simulink model "case1"  (R2024b)
settings: Solver=FixedStepAuto  StartTime=0  StopTime=1  FixedStep=1e-7  RelTol=1e-3
values from neighbouring files (symbols this model uses):
  SG_D_1_D = 0.01056    [IEEE9_case_parameters.m]    (also in case1_parameters.m; case2_parameters.m; case3_parameters.m; case4_parameters.m)
  SG_D_1_EnableSaturation = 0    [IEEE9_case_parameters.m]    (also in case1_parameters.m; case2_parameters.m; case3_parameters.m; case4_parameters.m)
  SG_D_1_f0 = 60    [IEEE9_case_parameters.m]    (also in case1_parameters.m; case2_parameters.m; case3_parameters.m; case4_parameters.m)
  SG_D_1_H = 7.5    [IEEE9_case_parameters.m]    (also in case1_parameters.m; case2_parameters.m; case3_parameters.m; case4_parameters.m)
  SG_D_1_K_A = 20    [IEEE9_case_parameters.m]    (also in case1_parameters.m; case2_parameters.m; case3_parameters.m; case4_parameters.m)
  SG_D_1_K_E = 1.000000e+1    (= 10)    [IEEE9_case_parameters.m]    (also in case1_parameters.m; case2_parameters.m; case3_parameters.m; case4_parameters.m)
  SG_D_1_K_F = 2.363    [IEEE9_case_parameters.m]    (also in case1_parameters.m; case2_parameters.m; case3_parameters.m; case4_parameters.m)
  SG_D_1_K_s = 0.5    [IEEE9_case_parameters.m]    (also in case1_parameters.m = 5; case2_parameters.m = 5; case3_parameters.m = 5; case4_parameters.m = 5)
  SG_D_1_R_a = 0.001088    [IEEE9_case_parameters.m]    (also in case1_parameters.m; case2_parameters.m; case3_parameters.m; case4_parameters.m)
  SG_D_1_S_A = 1    [IEEE9_case_parameters.m]    (also in case1_parameters.m; case2_parameters.m; case3_parameters.m; case4_parameters.m)
  SG_D_1_S_B = 0.103    [IEEE9_case_parameters.m]    (also in case1_parameters.m; case2_parameters.m; case3_parameters.m; case4_parameters.m)
  SG_D_1_S_N = 10.659857    [IEEE9_case_parameters.m]    (also in case1_parameters.m; case2_parameters.m; case3_parameters.m; case4_parameters.m)
  SG_D_1_SpeedPara = 200    [IEEE9_case_parameters.m]    (also in case1_parameters.m; case2_parameters.m; case3_parameters.m; case4_parameters.m)
  SG_D_1_T_0 = 0.720173    [IEEE9_case_parameters.m]    (also in case1_parameters.m = 0.755522; case2_parameters.m = 0.808931; case3_parameters.m = 0.869402; case4_parameters.m = 0.729316)
  SG_D_1_T_1 = 0.3    [IEEE9_case_parameters.m]    (also in case1_parameters.m; case2_parameters.m; case3_parameters.m; case4_parameters.m)
  SG_D_1_T_2 = 0.05    [IEEE9_case_parameters.m]    (also in case1_parameters.m; case2_parameters.m; case3_parameters.m; case4_parameters.m)
  SG_D_1_T_3 = 0.02    [IEEE9_case_parameters.m]    (also in case1_parameters.m; case2_parameters.m; case3_parameters.m; case4_parameters.m)
  SG_D_1_T_4 = 0.005    [IEEE9_case_parameters.m]    (also in case1_parameters.m; case2_parameters.m; case3_parameters.m; case4_parameters.m)
  SG_D_1_T_A = 0.02    [IEEE9_case_parameters.m]    (also in case1_parameters.m; case2_parameters.m; case3_parameters.m; case4_parameters.m)
  SG_D_1_T_dd = 8.000000e+0    (= 8)    [IEEE9_case_parameters.m]    (also in case1_parameters.m; case2_parameters.m; case3_parameters.m; case4_parameters.m)
  SG_D_1_T_ddd = 0.04    [IEEE9_case_parameters.m]    (also in case1_parameters.m; case2_parameters.m; case3_parameters.m; case4_parameters.m)
  SG_D_1_T_E = 0.314    [IEEE9_case_parameters.m]    (also in case1_parameters.m; case2_parameters.m; case3_parameters.m; case4_parameters.m)
  SG_D_1_T_F = 0.35    [IEEE9_case_parameters.m]    (also in case1_parameters.m; case2_parameters.m; case3_parameters.m; case4_parameters.m)
  SG_D_1_T_qd = 0.8    [IEEE9_case_parameters.m]    (also in case1_parameters.m; case2_parameters.m; case3_parameters.m; case4_parameters.m)
  SG_D_1_T_qdd = 0.02    [IEEE9_case_parameters.m]    (also in case1_parameters.m; case2_parameters.m; case3_parameters.m; case4_parameters.m)
  SG_D_1_T_speed = 0.1    [IEEE9_case_parameters.m]    (also in case1_parameters.m = 200; case2_parameters.m = 200; case3_parameters.m = 200; case4_parameters.m = 200)
  SG_D_1_T_w = 0.5    [IEEE9_case_parameters.m]    (also in case1_parameters.m; case2_parameters.m; case3_parameters.m; case4_parameters.m)
  SG_D_1_V_ref = 1.990276    [IEEE9_case_parameters.m]    (also in case1_parameters.m = 2.042296; case2_parameters.m = 2.051388; case3_parameters.m = 2.089584; case4_parameters.m = 2.01845)
  SG_D_1_w_ref = 376.991118    [IEEE9_case_parameters.m]    (also in case1_parameters.m; case2_parameters.m; case3_parameters.m; case4_parameters.m)
  SG_D_1_wb = 6.000000e+1    (= 60)    [IEEE9_case_parameters.m]    (also in case1_parameters.m; case2_parameters.m; case3_parameters.m; case4_parameters.m)
  SG_D_1_x_d = 1.9    [IEEE9_case_parameters.m]    (also in case1_parameters.m; case2_parameters.m; case3_parameters.m; case4_parameters.m)
  SG_D_1_x_dd = 0.302    [IEEE9_case_parameters.m]    (also in case1_parameters.m; case2_parameters.m; case3_parameters.m; case4_parameters.m)
  SG_D_1_x_ddd = 0.204    [IEEE9_case_parameters.m]    (also in case1_parameters.m; case2_parameters.m; case3_parameters.m; case4_parameters.m)
  SG_D_1_x_l = 0.05    [IEEE9_case_parameters.m]    (also in case1_parameters.m; case2_parameters.m; case3_parameters.m; case4_parameters.m)
  SG_D_1_x_q = 1.3    [IEEE9_case_parameters.m]    (also in case1_parameters.m; case2_parameters.m; case3_parameters.m; case4_parameters.m)
  SG_D_1_x_qd = 0.5    [IEEE9_case_parameters.m]    (also in case1_parameters.m; case2_parameters.m; case3_parameters.m; case4_parameters.m)
  SG_D_1_x_qdd = 0.3    [IEEE9_case_parameters.m]    (also in case1_parameters.m; case2_parameters.m; case3_parameters.m; case4_parameters.m)
  SG_D_2_D = 0.02    [IEEE9_case_parameters.m]    (also in case1_parameters.m; case2_parameters.m; case3_parameters.m; case4_parameters.m)
  SG_D_2_EnableSaturation = 0    [IEEE9_case_parameters.m]    (also in case1_parameters.m; case2_parameters.m; case3_parameters.m; case4_parameters.m)
  SG_D_2_f0 = 60    [IEEE9_case_parameters.m]    (also in case1_parameters.m; case2_parameters.m; case3_parameters.m; case4_parameters.m)
  SG_D_2_H = 8.000000e+0    (= 8)    [IEEE9_case_parameters.m]    (also in case1_parameters.m; case2_parameters.m; case3_parameters.m; case4_parameters.m)
  SG_D_2_K_A = 20    [IEEE9_case_parameters.m]    (also in case1_parameters.m; case2_parameters.m; case3_parameters.m; case4_parameters.m)
  SG_D_2_K_E = 1.000000e+1    (= 10)    [IEEE9_case_parameters.m]    (also in case1_parameters.m; case2_parameters.m; case3_parameters.m; case4_parameters.m)
  SG_D_2_K_F = 2.363    [IEEE9_case_parameters.m]    (also in case1_parameters.m; case2_parameters.m; case3_parameters.m; case4_parameters.m)
  SG_D_2_K_s = 0.5    [IEEE9_case_parameters.m]    (also in case1_parameters.m = 4; case2_parameters.m = 4; case3_parameters.m = 4; case4_parameters.m = 4)
  SG_D_2_R_a = 0.001088    [IEEE9_case_parameters.m]    (also in case1_parameters.m; case2_parameters.m; case3_parameters.m; case4_parameters.m)
  SG_D_2_S_A = 1    [IEEE9_case_parameters.m]    (also in case1_parameters.m; case2_parameters.m; case3_parameters.m; case4_parameters.m)
  SG_D_2_S_B = 0.103    [IEEE9_case_parameters.m]    (also in case1_parameters.m; case2_parameters.m; case3_parameters.m; case4_parameters.m)
  SG_D_2_S_N = 10.659857    [IEEE9_case_parameters.m]    (also in case1_parameters.m; case2_parameters.m; case3_parameters.m; case4_parameters.m)
  SG_D_2_SpeedPara = 200    [IEEE9_case_parameters.m]    (also in case1_parameters.m; case2_parameters.m; case3_parameters.m; case4_parameters.m)
  SG_D_2_T_0 = 1.632913    [IEEE9_case_parameters.m]    (also in case1_parameters.m = 1.632925; case2_parameters.m = 1.632915; case3_parameters.m = 1.632914; case4_parameters.m = 1.632927)
  SG_D_2_T_1 = 0.2    [IEEE9_case_parameters.m]    (also in case1_parameters.m; case2_parameters.m; case3_parameters.m; case4_parameters.m)
  SG_D_2_T_2 = 0.05    [IEEE9_case_parameters.m]    (also in case1_parameters.m; case2_parameters.m; case3_parameters.m; case4_parameters.m)
  SG_D_2_T_3 = 0.02    [IEEE9_case_parameters.m]    (also in case1_parameters.m; case2_parameters.m; case3_parameters.m; case4_parameters.m)
  SG_D_2_T_4 = 0.005    [IEEE9_case_parameters.m]    (also in case1_parameters.m; case2_parameters.m; case3_parameters.m; case4_parameters.m)
  SG_D_2_T_A = 0.02    [IEEE9_case_parameters.m]    (also in case1_parameters.m; case2_parameters.m; case3_parameters.m; case4_parameters.m)
  SG_D_2_T_dd = 7.9    [IEEE9_case_parameters.m]    (also in case1_parameters.m; case2_parameters.m; case3_parameters.m; case4_parameters.m)
  SG_D_2_T_ddd = 0.04    [IEEE9_case_parameters.m]    (also in case1_parameters.m; case2_parameters.m; case3_parameters.m; case4_parameters.m)
  SG_D_2_T_E = 0.314    [IEEE9_case_parameters.m]    (also in case1_parameters.m; case2_parameters.m; case3_parameters.m; case4_parameters.m)
  SG_D_2_T_F = 0.35    [IEEE9_case_parameters.m]    (also in case1_parameters.m; case2_parameters.m; case3_parameters.m; case4_parameters.m)
  SG_D_2_T_qd = 0.8    [IEEE9_case_parameters.m]    (also in case1_parameters.m; case2_parameters.m; case3_parameters.m; case4_parameters.m)
  SG_D_2_T_qdd = 0.015    [IEEE9_case_parameters.m]    (also in case1_parameters.m; case2_parameters.m; case3_parameters.m; case4_parameters.m)
  SG_D_2_T_speed = 0.1    [IEEE9_case_parameters.m]    (also in case1_parameters.m = 150; case2_parameters.m = 150; case3_parameters.m = 150; case4_parameters.m = 150)
  SG_D_2_T_w = 0.35    [IEEE9_case_parameters.m]    (also in case1_parameters.m; case2_parameters.m; case3_parameters.m; case4_parameters.m)
  SG_D_2_V_ref = 2.58547    [IEEE9_case_parameters.m]    (also in case1_parameters.m = 2.597896; case2_parameters.m = 2.587136; case3_parameters.m = 2.586042; case4_parameters.m = 2.599679)
  SG_D_2_w_ref = 376.991118    [IEEE9_case_parameters.m]    (also in case1_parameters.m; case2_parameters.m; case3_parameters.m; case4_parameters.m)
  SG_D_2_wb = 6.000000e+1    (= 60)    [IEEE9_case_parameters.m]    (also in case1_parameters.m; case2_parameters.m; case3_parameters.m; case4_parameters.m)
  SG_D_2_x_d = 1.8    [IEEE9_case_parameters.m]    (also in case1_parameters.m; case2_parameters.m; case3_parameters.m; case4_parameters.m)
  SG_D_2_x_dd = 0.302    [IEEE9_case_parameters.m]    (also in case1_parameters.m; case2_parameters.m; case3_parameters.m; case4_parameters.m)
  SG_D_2_x_ddd = 0.204    [IEEE9_case_parameters.m]    (also in case1_parameters.m; case2_parameters.m; case3_parameters.m; case4_parameters.m)
  SG_D_2_x_l = 0.05    [IEEE9_case_parameters.m]    (also in case1_parameters.m; case2_parameters.m; case3_parameters.m; case4_parameters.m)
  SG_D_2_x_q = 1.25    [IEEE9_case_parameters.m]    (also in case1_parameters.m; case2_parameters.m; case3_parameters.m; case4_parameters.m)
  SG_D_2_x_qd = 0.5    [IEEE9_case_parameters.m]    (also in case1_parameters.m; case2_parameters.m; case3_parameters.m; case4_parameters.m)
  SG_D_2_x_qdd = 0.3    [IEEE9_case_parameters.m]    (also in case1_parameters.m; case2_parameters.m; case3_parameters.m; case4_parameters.m)
  SG_D_3_D = 0.02    [IEEE9_case_parameters.m]    (also in case1_parameters.m; case2_parameters.m; case3_parameters.m; case4_parameters.m)
  SG_D_3_EnableSaturation = 0    [IEEE9_case_parameters.m]    (also in case1_parameters.m; case2_parameters.m; case3_parameters.m; case4_parameters.m)
  SG_D_3_f0 = 60    [IEEE9_case_parameters.m]    (also in case1_parameters.m; case2_parameters.m; case3_parameters.m; case4_parameters.m)
  SG_D_3_H = 7.7    [IEEE9_case_parameters.m]    (also in case1_parameters.m; case2_parameters.m; case3_parameters.m; case4_parameters.m)
  SG_D_3_K_A = 20    [IEEE9_case_parameters.m]    (also in case1_parameters.m; case2_parameters.m; case3_parameters.m; case4_parameters.m)
  SG_D_3_K_E = 1.000000e+1    (= 10)    [IEEE9_case_parameters.m]    (also in case1_parameters.m; case2_parameters.m; case3_parameters.m; case4_parameters.m)
  SG_D_3_K_F = 2.363    [IEEE9_case_parameters.m]    (also in case1_parameters.m; case2_parameters.m; case3_parameters.m; case4_parameters.m)
  SG_D_3_K_s = 0.2    [IEEE9_case_parameters.m]    (also in case1_parameters.m = 2; case2_parameters.m = 2; case3_parameters.m = 2; case4_parameters.m = 2)
  SG_D_3_R_a = 0.001088    [IEEE9_case_parameters.m]    (also in case1_parameters.m; case2_parameters.m; case3_parameters.m; case4_parameters.m)
  SG_D_3_S_A = 1    [IEEE9_case_parameters.m]    (also in case1_parameters.m; case2_parameters.m; case3_parameters.m; case4_parameters.m)
  SG_D_3_S_B = 0.103    [IEEE9_case_parameters.m]    (also in case1_parameters.m; case2_parameters.m; case3_parameters.m; case4_parameters.m)
  SG_D_3_S_N = 10.659857    [IEEE9_case_parameters.m]    (also in case1_parameters.m; case2_parameters.m; case3_parameters.m; case4_parameters.m)
  SG_D_3_SpeedPara = 200    [IEEE9_case_parameters.m]    (also in case1_parameters.m; case2_parameters.m; case3_parameters.m; case4_parameters.m)
  SG_D_3_T_0 = 0.850788    [IEEE9_case_parameters.m]    (also in case1_parameters.m = 0.850786; case2_parameters.m = 0.850787; case3_parameters.m; case4_parameters.m = 0.850786)
  SG_D_3_T_1 = 0.2    [IEEE9_case_parameters.m]    (also in case1_parameters.m; case2_parameters.m; case3_parameters.m; case4_parameters.m)
  SG_D_3_T_2 = 0.05    [IEEE9_case_parameters.m]    (also in case1_parameters.m; case2_parameters.m; case3_parameters.m; case4_parameters.m)
  SG_D_3_T_3 = 0.02    [IEEE9_case_parameters.m]    (also in case1_parameters.m; case2_parameters.m; case3_parameters.m; case4_parameters.m)
  SG_D_3_T_4 = 0.005    [IEEE9_case_parameters.m]    (also in case1_parameters.m; case2_parameters.m; case3_parameters.m; case4_parameters.m)
  SG_D_3_T_A = 0.02    [IEEE9_case_parameters.m]    (also in case1_parameters.m; case2_parameters.m; case3_parameters.m; case4_parameters.m)
  SG_D_3_T_dd = 8.1    [IEEE9_case_parameters.m]    (also in case1_parameters.m; case2_parameters.m; case3_parameters.m; case4_parameters.m)
  SG_D_3_T_ddd = 0.04    [IEEE9_case_parameters.m]    (also in case1_parameters.m; case2_parameters.m; case3_parameters.m; case4_parameters.m)
  SG_D_3_T_E = 0.314    [IEEE9_case_parameters.m]    (also in case1_parameters.m; case2_parameters.m; case3_parameters.m; case4_parameters.m)
  SG_D_3_T_F = 0.35    [IEEE9_case_parameters.m]    (also in case1_parameters.m; case2_parameters.m; case3_parameters.m; case4_parameters.m)
  SG_D_3_T_qd = 0.8    [IEEE9_case_parameters.m]    (also in case1_parameters.m; case2_parameters.m; case3_parameters.m; case4_parameters.m)
  SG_D_3_T_qdd = 0.015    [IEEE9_case_parameters.m]    (also in case1_parameters.m; case2_parameters.m; case3_parameters.m; case4_parameters.m)
  SG_D_3_T_speed = 0.1    [IEEE9_case_parameters.m]    (also in case1_parameters.m = 180; case2_parameters.m = 180; case3_parameters.m = 180; case4_parameters.m = 180)
  SG_D_3_T_w = 0.4    [IEEE9_case_parameters.m]    (also in case1_parameters.m; case2_parameters.m; case3_parameters.m; case4_parameters.m)
  SG_D_3_V_ref = 1.892727    [IEEE9_case_parameters.m]    (also in case1_parameters.m = 1.906439; case2_parameters.m = 1.895535; case3_parameters.m = 1.892105; case4_parameters.m = 1.906598)
  SG_D_3_w_ref = 376.991118    [IEEE9_case_parameters.m]    (also in case1_parameters.m; case2_parameters.m; case3_parameters.m; case4_parameters.m)
  SG_D_3_wb = 6.000000e+1    (= 60)    [IEEE9_case_parameters.m]    (also in case1_parameters.m; case2_parameters.m; case3_parameters.m; case4_parameters.m)
  SG_D_3_x_d = 1.85    [IEEE9_case_parameters.m]    (also in case1_parameters.m; case2_parameters.m; case3_parameters.m; case4_parameters.m)
  SG_D_3_x_dd = 0.302    [IEEE9_case_parameters.m]    (also in case1_parameters.m; case2_parameters.m; case3_parameters.m; case4_parameters.m)
  SG_D_3_x_ddd = 0.204    [IEEE9_case_parameters.m]    (also in case1_parameters.m; case2_parameters.m; case3_parameters.m; case4_parameters.m)
  SG_D_3_x_l = 0.05    [IEEE9_case_parameters.m]    (also in case1_parameters.m; case2_parameters.m; case3_parameters.m; case4_parameters.m)
  SG_D_3_x_q = 1.2    [IEEE9_case_parameters.m]    (also in case1_parameters.m; case2_parameters.m; case3_parameters.m; case4_parameters.m)
  SG_D_3_x_qd = 0.5    [IEEE9_case_parameters.m]    (also in case1_parameters.m; case2_parameters.m; case3_parameters.m; case4_parameters.m)
  SG_D_3_x_qdd = 0.3    [IEEE9_case_parameters.m]    (also in case1_parameters.m; case2_parameters.m; case3_parameters.m; case4_parameters.m)
(part 10 of 12)

== system case1/SG_D_3/d_R_f_SG_D_3_block ==
  note: d_R_f_SG_D_3 in case1
      | $-\frac{R_{f,\mathrm{SG},D,3}-\frac{E_{\mathrm{fd},\mathrm{SG},D,3}\,K_{F}}{T_{F}}}{T_{F}}$
      | Automatically generated on 2025-10-31 18:49:57 .
  State_E_fd_SG_D_3_666b5 : Inport
  State_R_f_SG_D_3_7f0e0 : Inport  Port=2
  Constant_K_F_3ac82 : Constant  Value=K_F
  Constant_T_F_aca80 : Constant  Value=T_F
  Constant_T_F_d3988 : Constant  Value=T_F
  Divide_c9ce7 : Product  Inputs=*/
  Divide_de91c : Product  Inputs=*/
  Product_63f86 : Product
  Subtract_163d8 : Sum  Inputs=+-
  Blockout_d_R_f_SG_D_3_113ff : Outport
  wires:
  State_E_fd_SG_D_3_666b5/1 -> Product_63f86/1
  Constant_T_F_d3988/1 -> Divide_c9ce7/2
  Constant_K_F_3ac82/1 -> Product_63f86/2
  Product_63f86/1 -> Divide_c9ce7/1
  Divide_c9ce7/1 -> Subtract_163d8/1
  State_R_f_SG_D_3_7f0e0/1 -> Subtract_163d8/2
  Subtract_163d8/1 -> Divide_de91c/1
  Constant_T_F_aca80/1 -> Divide_de91c/2
  Divide_de91c/1 -> Blockout_d_R_f_SG_D_3_113ff/1

== system case1/SG_D_3/d_T_m_SG_D_3_block ==
  note: d_T_m_SG_D_3 in case1
      | $-\frac{T_{m,\mathrm{SG},D,3}-T_{0}+\frac{\mathrm{SpeedPara}\,\left(w_{\mathrm{SG},D,3}-w_{\mathrm{ref}}\right)}{2\,f_{0}\,\pi }}{T_{\mathrm{speed}}}$
      | Automatically generated on 2025-10-31 18:49:52 .
  State_w_SG_D_3_66142 : Inport
  State_T_m_SG_D_3_24b45 : Inport  Port=2
  Add_9f440 : Sum
  Add_ee289 : Sum
  Constant_-1_aa800 : Constant  Value=-1
  Constant_2.0_3da56 : Constant  Value=2.0
  Constant_SpeedPara_331ce : Constant  Value=SpeedPara
  Constant_T_0_ffd13 : Constant  Value=T_0
  Constant_T_speed_afd64 : Constant  Value=T_speed
  Constant_f0_5ced1 : Constant  Value=f0
  Constant_pi_16505 : Constant  Value=pi
  Constant_w_ref_a248d : Constant  Value=w_ref
  Divide_01cbf : Product  Inputs=*/
  Divide_61cdb : Product  Inputs=*/
  Product_7fe71 : Product
  Product_98dfd : Product
  Product_bc562 : Product
  Product_c22a6 : Product
  Subtract_d9e42 : Sum  Inputs=+-
  Blockout_d_T_m_SG_D_3_67a05 : Outport
  wires:
  Constant_SpeedPara_331ce/1 -> Product_7fe71/1
  Constant_-1_aa800/1 -> Product_98dfd/1
  Constant_w_ref_a248d/1 -> Add_9f440/2
  State_w_SG_D_3_66142/1 -> Product_98dfd/2
  Constant_2.0_3da56/1 -> Product_c22a6/1
  Product_98dfd/1 -> Add_9f440/1
  Constant_pi_16505/1 -> Product_c22a6/2
  Add_9f440/1 -> Product_7fe71/2
  Product_c22a6/1 -> Product_bc562/1
  Constant_f0_5ced1/1 -> Product_bc562/2
  Product_7fe71/1 -> Divide_01cbf/1
  Product_bc562/1 -> Divide_01cbf/2
  Divide_01cbf/1 -> Add_ee289/1
  Constant_T_0_ffd13/1 -> Add_ee289/2
  Add_ee289/1 -> Subtract_d9e42/1
  State_T_m_SG_D_3_24b45/1 -> Subtract_d9e42/2
  Subtract_d9e42/1 -> Divide_61cdb/1
  Constant_T_speed_afd64/1 -> Divide_61cdb/2
  Divide_61cdb/1 -> Blockout_d_T_m_SG_D_3_67a05/1

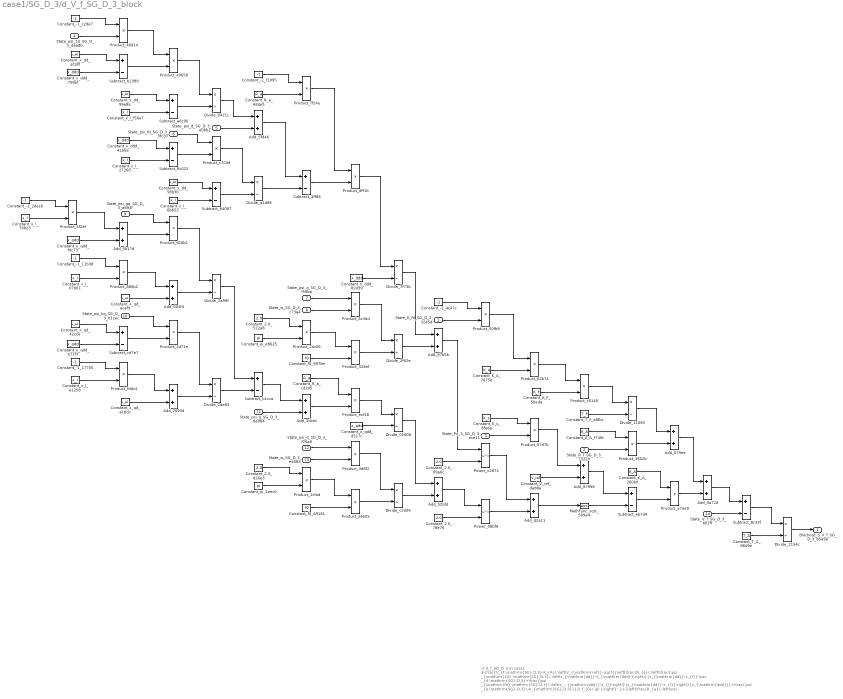
== system case1/SG_D_3/d_V_f_SG_D_3_block ==
  note: d_V_f_SG_D_3 in case1
      | $-\frac{V_{f,\mathrm{SG},D,3}-K_{A}\,\left(V_{\mathrm{ref}}-\sqrt{{\left(\frac{R_{a}\,\left(\frac{\psi _{\mathrm{1d},\mathrm{SG},D,3}\,\left(x_{\mathrm{dd}}-x_{\mathrm{ddd}}\right)}{x_{\mathrm{dd}}-x_{l}}-\psi _{d,\mathrm{SG},D,3}+\frac{\psi _{\mathrm{fd},\mathrm{SG},D,3}\,\left(x_{\mathrm{ddd}}-x_{l}\right)}{x_{\mathrm{dd}}-x_{l}}\right)}{x_{\mathrm{ddd}}}+\frac{\psi _{q,\mathrm{SG},D,3}\,w_{\mathrm{SG},D,3}}{2\,f_{0}\,\pi }\right)}^2+{\left(\frac{R_{a}\,\left(\psi _{q,\mathrm{SG},D,3}+\frac{\psi _{\mathrm{gq},\mathrm{SG},D,3}\,\left(x_{l}-x_{\mathrm{qdd}}\right)}{x_{l}-x_{\mathrm{qd}}}+\frac{\psi _{\mathrm{kq},\mathrm{SG},D,3}\,\left(x_{\mathrm{qd}}-x_{\mathrm{qdd}}\right)}{x_{l}-x_{\mathrm{qd}}}\right)}{x_{\mathrm{qdd}}}+\frac{\psi _{d,\mathrm{SG},D,3}\,w_{\mathrm{SG},D,3}}{2\,f_{0}\,\pi }\right)}^2}+K_{s}\,\mathrm{Px}_{3,\mathrm{SG},D,3}\right)-K_{A}\,R_{f,\mathrm{SG},D,3}+\frac{E_{\mathrm{fd},\mathrm{SG},D,3}\,K_{A}\,K_{F}}{T_{F}}}{T_{A}}$
      | Automatically generated on 2025-10-31 18:49:56 .
  State_E_fd_SG_D_3_3245d : Inport
  State_R_f_SG_D_3_73220 : Inport  Port=2
  State_Px_3_SG_D_3_ece11 : Inport  Port=3
  State_psi_1d_SG_D_3_daa8b : Inport  Port=4
  State_psi_d_SG_D_3_e0bb1 : Inport  Port=5
  State_psi_fd_SG_D_3_3fc20 : Inport  Port=6
  State_psi_q_SG_D_3_f59ba : Inport  Port=7
  State_w_SG_D_3_c73a4 : Inport  Port=8
  State_psi_gq_SG_D_3_a694f : Inport  Port=9
  State_psi_kq_SG_D_3_b1cec : Inport  Port=10
  State_psi_q_SG_D_3_dedb4 : Inport  Port=11
  State_psi_d_SG_D_3_f76a9 : Inport  Port=12
  State_w_SG_D_3_e4083 : Inport  Port=13
  State_V_f_SG_D_3_b01ff : Inport  Port=14
  Add_079ee : Sum
  Add_0a72d : Sum
  Add_2093d : Sum
  Add_3dcec : Sum
  Add_52bfd : Sum
  Add_5b17d : Sum
  Add_5fd46 : Sum
  Add_604f4 : Sum
  Add_87996 : Sum
  Add_97b5b : Sum
  Add_d2a11 : Sum
  Constant_-1_11b38 : Constant  Value=-1
  Constant_-1_17705 : Constant  Value=-1
  Constant_-1_2decb : Constant  Value=-1
  Constant_-1_4c47c : Constant  Value=-1
  Constant_-1_c29e7 : Constant  Value=-1
  Constant_-1_f1995 : Constant  Value=-1
  Constant_2.0_09a6c : Constant  Value=2.0
  Constant_2.0_522a8 : Constant  Value=2.0
  Constant_2.0_78e76 : Constant  Value=2.0
  Constant_2.0_d26e3 : Constant  Value=2.0
  Constant_K_A_260b0 : Constant  Value=K_A
  Constant_K_A_7675b : Constant  Value=K_A
  Constant_K_A_f74fe : Constant  Value=K_A
  Constant_K_F_50eda : Constant  Value=K_F
  Constant_K_s_8fe6a : Constant  Value=K_s
  Constant_R_a_68de5 : Constant  Value=R_a
  Constant_R_a_cd2d5 : Constant  Value=R_a
  Constant_T_A_8849e : Constant  Value=T_A
  Constant_T_F_af8bc : Constant  Value=T_F
  Constant_V_ref_da88a : Constant  Value=V_ref
  Constant_f0_69181 : Constant  Value=f0
  Constant_f0_9978e : Constant  Value=f0
  Constant_pi_1eec0 : Constant  Value=pi
  Constant_pi_e8625 : Constant  Value=pi
  Constant_x_dd_58b30 : Constant  Value=x_dd
  Constant_x_dd_99e8a : Constant  Value=x_dd
  Constant_x_dd_af18f : Constant  Value=x_dd
  Constant_x_ddd_41b5a : Constant  Value=x_ddd
  Constant_x_ddd_758ef : Constant  Value=x_ddd
  Constant_x_ddd_82d39 : Constant  Value=x_ddd
  Constant_x_l_07001 : Constant  Value=x_l
  Constant_x_l_27260 : Constant  Value=x_l
  Constant_x_l_6b652 : Constant  Value=x_l
  Constant_x_l_79823 : Constant  Value=x_l
  Constant_x_l_e1258 : Constant  Value=x_l
  Constant_x_l_f56a7 : Constant  Value=x_l
  Constant_x_qd_42cce : Constant  Value=x_qd
  Constant_x_qd_a18cb : Constant  Value=x_qd
  Constant_x_qd_acaf9 : Constant  Value=x_qd
  Constant_x_qdd_d517c : Constant  Value=x_qdd
  Constant_x_qdd_e71f3 : Constant  Value=x_qdd
  Constant_x_qdd_fdc73 : Constant  Value=x_qdd
  Divide_01608 : Product  Inputs=*/
  Divide_11083 : Product  Inputs=*/
  Divide_2154c : Product  Inputs=*/
  Divide_2a99f : Product  Inputs=*/
  Divide_2de83 : Product  Inputs=*/
  Divide_2f62e : Product  Inputs=*/
  Divide_7f73b : Product  Inputs=*/
  Divide_9421c : Product  Inputs=*/
  Divide_a1d88 : Product  Inputs=*/
  Divide_c2d09 : Product  Inputs=*/
  MathFunc_sqrt_599a4 : Sqrt
  Power_08bf6 : Math  Operator=pow
  Power_c2873 : Math  Operator=pow
  Product_1cfad : Product
  Product_26a05 : Product
  Product_2d71e : Product
  Product_2dc06 : Product
  Product_328ef : Product
  Product_3802b : Product
  Product_3d8f2 : Product
  Product_46914 : Product
  Product_4f2af : Product
  Product_50fb9 : Product
  Product_62b74 : Product
  Product_67d7b : Product
  Product_6c3dd : Product
  Product_880b2 : Product
  Product_a0658 : Product
  Product_a7ae9 : Product
  Product_c0148 : Product
  Product_c703d : Product
  Product_d16b1 : Product
  Product_dff1b : Product
  Product_ecf18 : Product
  Product_fddc4 : Product
  Product_ff24e : Product
  Subtract_4ff88 : Sum  Inputs=+-
  Subtract_64097 : Sum  Inputs=+-
  Subtract_8c022 : Sum  Inputs=+-
  Subtract_8c33f : Sum  Inputs=+-
  Subtract_a6c00 : Sum  Inputs=+-
  Subtract_b1cca : Sum  Inputs=+-
  Subtract_b2389 : Sum  Inputs=+-
  Subtract_cd7e7 : Sum  Inputs=+-
  Subtract_eb7d4 : Sum  Inputs=+-
  Blockout_d_V_f_SG_D_3_85a9a : Outport
  wires:
  Constant_K_A_f74fe/1 -> Product_3802b/1
  Constant_-1_2decb/1 -> Product_4f2af/1
  Subtract_8c022/1 -> Product_c703d/2
  Constant_x_l_79823/1 -> Product_4f2af/2
  Divide_c2d09/1 -> Add_52bfd/2
  Constant_-1_c29e7/1 -> Product_46914/1
  State_psi_1d_SG_D_3_daa8b/1 -> Product_46914/2
  Constant_x_dd_af18f/1 -> Subtract_b2389/1
  Divide_a1d88/1 -> Subtract_4ff88/2
  Product_4f2af/1 -> Add_5b17d/1
  Constant_x_qdd_fdc73/1 -> Add_5b17d/2
  Constant_x_ddd_758ef/1 -> Subtract_b2389/2
  Constant_2.0_78e76/1 -> Power_08bf6/2
  Constant_-1_11b38/1 -> Product_880b2/1
  Divide_2a99f/1 -> Subtract_b1cca/1
  Subtract_a6c00/1 -> Divide_9421c/2
  Constant_x_l_07001/1 -> Product_880b2/2
  Constant_x_qd_42cce/1 -> Subtract_cd7e7/1
  State_w_SG_D_3_c73a4/1 -> Product_6c3dd/2
  Constant_x_qdd_e71f3/1 -> Subtract_cd7e7/2
  Constant_2.0_522a8/1 -> Product_2dc06/1
  Constant_-1_17705/1 -> Product_fddc4/1
  Constant_pi_e8625/1 -> Product_2dc06/2
  Add_5fd46/1 -> Subtract_4ff88/1
  Constant_x_l_e1258/1 -> Product_fddc4/2
  Product_46914/1 -> Product_a0658/1
  Subtract_b2389/1 -> Product_a0658/2
  Constant_2.0_d26e3/1 -> Product_1cfad/1
  Constant_x_dd_99e8a/1 -> Subtract_a6c00/1
  Constant_pi_1eec0/1 -> Product_1cfad/2
  Constant_x_l_f56a7/1 -> Subtract_a6c00/2
  Constant_x_ddd_41b5a/1 -> Subtract_8c022/1
  Constant_x_l_27260/1 -> Subtract_8c022/2
  State_psi_gq_SG_D_3_a694f/1 -> Product_d16b1/1
  Constant_x_l_6b652/1 -> Subtract_64097/2
  Add_5b17d/1 -> Product_d16b1/2
  Product_880b2/1 -> Add_604f4/1
  Product_d16b1/1 -> Divide_2a99f/1
  Constant_x_qd_acaf9/1 -> Add_604f4/2
  State_psi_kq_SG_D_3_b1cec/1 -> Product_2d71e/1
  State_psi_q_SG_D_3_f59ba/1 -> Product_6c3dd/1
  Add_97b5b/1 -> Power_c2873/1
  Subtract_cd7e7/1 -> Product_2d71e/2
  Constant_f0_9978e/1 -> Product_328ef/2
  Product_2dc06/1 -> Product_328ef/1
  Constant_x_qd_a18cb/1 -> Add_2093d/2
  Product_fddc4/1 -> Add_2093d/1
  Product_a0658/1 -> Divide_9421c/1
  State_psi_fd_SG_D_3_3fc20/1 -> Product_c703d/1
  Constant_x_dd_58b30/1 -> Subtract_64097/1
  Add_604f4/1 -> Divide_2a99f/2
  Add_d2a11/1 -> MathFunc_sqrt_599a4/1
  Product_2d71e/1 -> Divide_2de83/1
  Add_2093d/1 -> Divide_2de83/2
  Product_ff24e/1 -> Product_dff1b/1
  Divide_9421c/1 -> Add_5fd46/1
  Add_87996/1 -> Subtract_eb7d4/1
  State_psi_d_SG_D_3_e0bb1/1 -> Add_5fd46/2
  Product_c703d/1 -> Divide_a1d88/1
  Subtract_64097/1 -> Divide_a1d88/2
  MathFunc_sqrt_599a4/1 -> Subtract_eb7d4/2
  Divide_2de83/1 -> Subtract_b1cca/2
  Constant_-1_f1995/1 -> Product_ff24e/1
  Constant_R_a_68de5/1 -> Product_ff24e/2
  Subtract_b1cca/1 -> Add_3dcec/1
  State_psi_q_SG_D_3_dedb4/1 -> Add_3dcec/2
  Subtract_4ff88/1 -> Product_dff1b/2
  Constant_R_a_cd2d5/1 -> Product_ecf18/1
  Add_3dcec/1 -> Product_ecf18/2
  State_psi_d_SG_D_3_f76a9/1 -> Product_3d8f2/1
  State_w_SG_D_3_e4083/1 -> Product_3d8f2/2
  Product_1cfad/1 -> Product_26a05/1
  Constant_f0_69181/1 -> Product_26a05/2
  Product_dff1b/1 -> Divide_7f73b/1
  Constant_x_ddd_82d39/1 -> Divide_7f73b/2
  Product_6c3dd/1 -> Divide_2f62e/1
  Product_328ef/1 -> Divide_2f62e/2
  Product_ecf18/1 -> Divide_01608/1
  Constant_x_qdd_d517c/1 -> Divide_01608/2
  Product_3d8f2/1 -> Divide_c2d09/1
  Product_26a05/1 -> Divide_c2d09/2
  Divide_7f73b/1 -> Add_97b5b/1
  Divide_2f62e/1 -> Add_97b5b/2
  Divide_01608/1 -> Add_52bfd/1
  Constant_-1_4c47c/1 -> Product_50fb9/1
  State_E_fd_SG_D_3_3245d/1 -> Product_50fb9/2
  Constant_2.0_09a6c/1 -> Power_c2873/2
  Add_52bfd/1 -> Power_08bf6/1
  Product_50fb9/1 -> Product_62b74/1
  Constant_K_A_7675b/1 -> Product_62b74/2
  Constant_K_s_8fe6a/1 -> Product_67d7b/1
  State_Px_3_SG_D_3_ece11/1 -> Product_67d7b/2
  Power_c2873/1 -> Add_d2a11/1
  Power_08bf6/1 -> Add_d2a11/2
  Product_62b74/1 -> Product_c0148/1
  Constant_K_F_50eda/1 -> Product_c0148/2
  Product_67d7b/1 -> Add_87996/1
  Constant_V_ref_da88a/1 -> Add_87996/2
  Product_c0148/1 -> Divide_11083/1
  Constant_T_F_af8bc/1 -> Divide_11083/2
  Add_0a72d/1 -> Subtract_8c33f/1
  State_R_f_SG_D_3_73220/1 -> Product_3802b/2
  Divide_11083/1 -> Add_079ee/1
  Product_3802b/1 -> Add_079ee/2
  Constant_K_A_260b0/1 -> Product_a7ae9/1
  Subtract_eb7d4/1 -> Product_a7ae9/2
  Add_079ee/1 -> Add_0a72d/1
  Product_a7ae9/1 -> Add_0a72d/2
  State_V_f_SG_D_3_b01ff/1 -> Subtract_8c33f/2
  Subtract_8c33f/1 -> Divide_2154c/1
  Constant_T_A_8849e/1 -> Divide_2154c/2
  Divide_2154c/1 -> Blockout_d_V_f_SG_D_3_85a9a/1

== system case1/SG_D_3/d_psi_1d_SG_D_3_block ==
  note: d_psi_1d_SG_D_3 in case1
      | $-\frac{\psi _{\mathrm{1d},\mathrm{SG},D,3}-\psi _{\mathrm{fd},\mathrm{SG},D,3}+\frac{\left(x_{\mathrm{dd}}-x_{l}\right)\,\left(\frac{\psi _{\mathrm{1d},\mathrm{SG},D,3}\,\left(x_{\mathrm{dd}}-x_{\mathrm{ddd}}\right)}{x_{\mathrm{dd}}-x_{l}}-\psi _{d,\mathrm{SG},D,3}+\frac{\psi _{\mathrm{fd},\mathrm{SG},D,3}\,\left(x_{\mathrm{ddd}}-x_{l}\right)}{x_{\mathrm{dd}}-x_{l}}\right)}{x_{\mathrm{ddd}}}}{T_{\mathrm{ddd}}}$
      | Automatically generated on 2025-10-31 18:49:34 .
  State_psi_1d_SG_D_3_697cb : Inport
  State_psi_fd_SG_D_3_10bdc : Inport  Port=2
  State_psi_1d_SG_D_3_13000 : Inport  Port=3
  State_psi_d_SG_D_3_fc886 : Inport  Port=4
  State_psi_fd_SG_D_3_12757 : Inport  Port=5
  Add_3cfcd : Sum
  Add_78f9b : Sum
  Add_d1ddf : Sum
  Constant_-1_a2fd8 : Constant  Value=-1
  Constant_-1_ded2b : Constant  Value=-1
  Constant_T_ddd_30346 : Constant  Value=T_ddd
  Constant_x_dd_19d87 : Constant  Value=x_dd
  Constant_x_dd_75615 : Constant  Value=x_dd
  Constant_x_dd_8bee4 : Constant  Value=x_dd
  Constant_x_dd_94806 : Constant  Value=x_dd
  Constant_x_ddd_00628 : Constant  Value=x_ddd
  Constant_x_ddd_bbd88 : Constant  Value=x_ddd
  Constant_x_ddd_d008a : Constant  Value=x_ddd
  Constant_x_l_28155 : Constant  Value=x_l
  Constant_x_l_85d91 : Constant  Value=x_l
  Constant_x_l_b1289 : Constant  Value=x_l
  Constant_x_l_d62ec : Constant  Value=x_l
  Divide_b8de5 : Product  Inputs=*/
  Divide_c2885 : Product  Inputs=*/
  Divide_d4862 : Product  Inputs=*/
  Divide_fcc5c : Product  Inputs=*/
  Product_59a27 : Product
  Product_7da4d : Product
  Product_83ab3 : Product
  Product_e3e48 : Product
  Product_e8351 : Product
  Subtract_09d84 : Sum  Inputs=+-
  Subtract_6d119 : Sum  Inputs=+-
  Subtract_9d6fb : Sum  Inputs=+-
  Subtract_e782b : Sum  Inputs=+-
  Subtract_f655b : Sum  Inputs=+-
  Subtract_fc28e : Sum  Inputs=+-
  Blockout_d_psi_1d_SG_D_3_1ecde : Outport
  wires:
  Divide_fcc5c/1 -> Add_3cfcd/1
  Subtract_09d84/1 -> Product_7da4d/2
  Constant_-1_a2fd8/1 -> Product_e3e48/1
  Constant_x_dd_19d87/1 -> Subtract_e782b/1
  State_psi_1d_SG_D_3_13000/1 -> Product_e3e48/2
  Product_e3e48/1 -> Product_7da4d/1
  Constant_x_dd_8bee4/1 -> Subtract_09d84/1
  Constant_x_ddd_d008a/1 -> Subtract_09d84/2
  Constant_x_l_b1289/1 -> Subtract_e782b/2
  Constant_x_ddd_00628/1 -> Subtract_6d119/1
  Divide_c2885/1 -> Blockout_d_psi_1d_SG_D_3_1ecde/1
  Constant_x_l_d62ec/1 -> Subtract_6d119/2
  Product_7da4d/1 -> Divide_fcc5c/1
  Subtract_e782b/1 -> Divide_fcc5c/2
  State_psi_fd_SG_D_3_12757/1 -> Product_83ab3/1
  Subtract_6d119/1 -> Product_83ab3/2
  Constant_x_dd_94806/1 -> Subtract_f655b/1
  Constant_x_l_28155/1 -> Subtract_f655b/2
  State_psi_d_SG_D_3_fc886/1 -> Add_3cfcd/2
  Product_83ab3/1 -> Divide_b8de5/1
  Subtract_f655b/1 -> Divide_b8de5/2
  Constant_x_dd_75615/1 -> Subtract_fc28e/1
  Constant_x_l_85d91/1 -> Subtract_fc28e/2
  Add_3cfcd/1 -> Subtract_9d6fb/1
  Divide_b8de5/1 -> Subtract_9d6fb/2
  Constant_-1_ded2b/1 -> Product_e8351/1
  State_psi_1d_SG_D_3_697cb/1 -> Product_e8351/2
  State_psi_fd_SG_D_3_10bdc/1 -> Add_78f9b/2
  Subtract_fc28e/1 -> Product_59a27/1
  Subtract_9d6fb/1 -> Product_59a27/2
  Product_e8351/1 -> Add_78f9b/1
  Product_59a27/1 -> Divide_d4862/1
  Constant_x_ddd_bbd88/1 -> Divide_d4862/2
  Add_78f9b/1 -> Add_d1ddf/1
  Divide_d4862/1 -> Add_d1ddf/2
  Add_d1ddf/1 -> Divide_c2885/1
  Constant_T_ddd_30346/1 -> Divide_c2885/2

== system case1/SG_D_3/d_psi_d_SG_D_3_block ==
  note: d_psi_d_SG_D_3 in case1
      | $2\,\pi \,f_{0}\,\left(v_{d,\mathrm{SG},D,3}\,\sin\left(\theta _{\mathrm{SG},D,3}\right)-v_{q,\mathrm{SG},D,3}\,\cos\left(\theta _{\mathrm{SG},D,3}\right)+\frac{R_{a}\,\left(\frac{\psi _{\mathrm{1d},\mathrm{SG},D,3}\,\left(x_{\mathrm{dd}}-x_{\mathrm{ddd}}\right)}{x_{\mathrm{dd}}-x_{l}}-\psi _{d,\mathrm{SG},D,3}+\frac{\psi _{\mathrm{fd},\mathrm{SG},D,3}\,\left(x_{\mathrm{ddd}}-x_{l}\right)}{x_{\mathrm{dd}}-x_{l}}\right)}{x_{\mathrm{ddd}}}+\frac{\psi _{q,\mathrm{SG},D,3}\,w_{\mathrm{SG},D,3}}{2\,f_{0}\,\pi }\right)$
      | Automatically generated on 2025-10-31 18:49:22 .
  State_psi_1d_SG_D_3_a5cf0 : Inport
  State_psi_d_SG_D_3_98be9 : Inport  Port=2
  State_psi_fd_SG_D_3_efb9b : Inport  Port=3
  Input_v_d_SG_D_3_1db53 : Inport  Port=4
  State_theta_SG_D_3_ff733 : Inport  Port=5
  Input_v_q_SG_D_3_da623 : Inport  Port=6
  State_theta_SG_D_3_0d41b : Inport  Port=7
  State_psi_q_SG_D_3_aaa02 : Inport  Port=8
  State_w_SG_D_3_2ec24 : Inport  Port=9
  Add_4f833 : Sum
  Add_b4f20 : Sum
  Constant_-1_f6838 : Constant  Value=-1
  Constant_-2.0_afe4f : Constant  Value=-2.0
  Constant_2.0_8818a : Constant  Value=2.0
  Constant_R_a_67289 : Constant  Value=R_a
  Constant_f0_0abb2 : Constant  Value=f0
  Constant_f0_4c223 : Constant  Value=f0
  Constant_pi_8a6e0 : Constant  Value=pi
  Constant_pi_94916 : Constant  Value=pi
  Constant_x_dd_20ce5 : Constant  Value=x_dd
  Constant_x_dd_980a3 : Constant  Value=x_dd
  Constant_x_dd_ad65b : Constant  Value=x_dd
  Constant_x_ddd_0de47 : Constant  Value=x_ddd
  Constant_x_ddd_6c376 : Constant  Value=x_ddd
  Constant_x_ddd_fa6fa : Constant  Value=x_ddd
  Constant_x_l_7caff : Constant  Value=x_l
  Constant_x_l_d815e : Constant  Value=x_l
  Constant_x_l_eb76f : Constant  Value=x_l
  Divide_5b586 : Product  Inputs=*/
  Divide_5bf52 : Product  Inputs=*/
  Divide_f238a : Product  Inputs=*/
  Divide_f89b0 : Product  Inputs=*/
  MathFunc_cos_535f4 : Trigonometry  Operator=cos
  MathFunc_sin_4ab83 : Trigonometry
  Product_25fc2 : Product
  Product_37ac0 : Product
  Product_54159 : Product
  Product_62209 : Product
  Product_692e6 : Product
  Product_7bde7 : Product
  Product_840e4 : Product
  Product_a93f5 : Product
  Product_b6921 : Product
  Product_c4393 : Product
  Product_c7cd5 : Product
  Product_d35ad : Product
  Subtract_081eb : Sum  Inputs=+-
  Subtract_0b52f : Sum  Inputs=+-
  Subtract_46979 : Sum  Inputs=+-
  Subtract_497c6 : Sum  Inputs=+-
  Subtract_9710f : Sum  Inputs=+-
  Subtract_997b8 : Sum  Inputs=+-
  Subtract_d05fc : Sum  Inputs=+-
  Blockout_d_psi_d_SG_D_3_cc8c1 : Outport
  wires:
  Constant_-1_f6838/1 -> Product_c4393/1
  Constant_2.0_8818a/1 -> Product_c7cd5/1
  Constant_x_dd_ad65b/1 -> Subtract_997b8/1
  State_psi_1d_SG_D_3_a5cf0/1 -> Product_c4393/2
  Constant_x_dd_20ce5/1 -> Subtract_9710f/1
  Constant_pi_94916/1 -> Product_c7cd5/2
  Constant_x_ddd_fa6fa/1 -> Subtract_997b8/2
  Product_c4393/1 -> Product_d35ad/1
  Product_c7cd5/1 -> Product_b6921/1
  Subtract_997b8/1 -> Product_d35ad/2
  Constant_-2.0_afe4f/1 -> Product_7bde7/1
  Constant_x_l_7caff/1 -> Subtract_9710f/2
  Constant_x_ddd_0de47/1 -> Subtract_497c6/1
  Constant_pi_8a6e0/1 -> Product_7bde7/2
  Constant_x_l_d815e/1 -> Subtract_497c6/2
  Product_54159/1 -> Divide_f89b0/1
  Product_d35ad/1 -> Divide_5b586/1
  Subtract_9710f/1 -> Divide_5b586/2
  State_psi_fd_SG_D_3_efb9b/1 -> Product_37ac0/1
  Subtract_497c6/1 -> Product_37ac0/2
  Constant_x_dd_980a3/1 -> Subtract_d05fc/1
  Constant_x_l_eb76f/1 -> Subtract_d05fc/2
  Divide_f89b0/1 -> Subtract_46979/2
  Divide_5b586/1 -> Add_4f833/1
  Subtract_081eb/1 -> Product_692e6/2
  State_psi_d_SG_D_3_98be9/1 -> Add_4f833/2
  Product_37ac0/1 -> Divide_5bf52/1
  Subtract_d05fc/1 -> Divide_5bf52/2
  Add_4f833/1 -> Subtract_081eb/1
  Divide_5bf52/1 -> Subtract_081eb/2
  Product_a93f5/1 -> Add_b4f20/2
  Constant_R_a_67289/1 -> Product_692e6/1
  Product_840e4/1 -> Product_62209/1
  State_theta_SG_D_3_ff733/1 -> MathFunc_sin_4ab83/1
  Product_692e6/1 -> Divide_f238a/1
  Constant_x_ddd_6c376/1 -> Divide_f238a/2
  Input_v_d_SG_D_3_1db53/1 -> Product_25fc2/1
  State_w_SG_D_3_2ec24/1 -> Product_54159/2
  MathFunc_sin_4ab83/1 -> Product_25fc2/2
  State_theta_SG_D_3_0d41b/1 -> MathFunc_cos_535f4/1
  MathFunc_cos_535f4/1 -> Product_a93f5/2
  Divide_f238a/1 -> Subtract_0b52f/1
  Product_25fc2/1 -> Subtract_0b52f/2
  Input_v_q_SG_D_3_da623/1 -> Product_a93f5/1
  State_psi_q_SG_D_3_aaa02/1 -> Product_54159/1
  Constant_f0_0abb2/1 -> Product_b6921/2
  Subtract_0b52f/1 -> Add_b4f20/1
  Product_b6921/1 -> Divide_f89b0/2
  Product_7bde7/1 -> Product_840e4/1
  Constant_f0_4c223/1 -> Product_840e4/2
  Add_b4f20/1 -> Subtract_46979/1
  Subtract_46979/1 -> Product_62209/2
  Product_62209/1 -> Blockout_d_psi_d_SG_D_3_cc8c1/1

== system case1/SG_D_3/d_psi_fd_SG_D_3_block ==
  note: d_psi_fd_SG_D_3 in case1
      | $-\frac{\psi _{\mathrm{fd},\mathrm{SG},D,3}-E_{\mathrm{fd},\mathrm{SG},D,3}+\left(x_{d}-x_{\mathrm{dd}}\right)\,\left(\frac{\frac{\psi _{\mathrm{1d},\mathrm{SG},D,3}\,\left(x_{\mathrm{dd}}-x_{\mathrm{ddd}}\right)}{x_{\mathrm{dd}}-x_{l}}-\psi _{d,\mathrm{SG},D,3}+\frac{\psi _{\mathrm{fd},\mathrm{SG},D,3}\,\left(x_{\mathrm{ddd}}-x_{l}\right)}{x_{\mathrm{dd}}-x_{l}}}{x_{\mathrm{ddd}}}-\frac{\left(x_{\mathrm{dd}}-x_{\mathrm{ddd}}\right)\,\left(\psi _{\mathrm{1d},\mathrm{SG},D,3}-\psi _{\mathrm{fd},\mathrm{SG},D,3}+\frac{\left(x_{\mathrm{dd}}-x_{l}\right)\,\left(\frac{\psi _{\mathrm{1d},\mathrm{SG},D,3}\,\left(x_{\mathrm{dd}}-x_{\mathrm{ddd}}\right)}{x_{\mathrm{dd}}-x_{l}}-\psi _{d,\mathrm{SG},D,3}+\frac{\psi _{\mathrm{fd},\mathrm{SG},D,3}\,\left(x_{\mathrm{ddd}}-x_{l}\right)}{x_{\mathrm{dd}}-x_{l}}\right)}{x_{\mathrm{ddd}}}\right)}{{\left(x_{\mathrm{dd}}-x_{l}\right)}^2}\right)}{T_{\mathrm{dd}}}$
      | Automatically generated on 2025-10-31 18:49:31 .
  State_E_fd_SG_D_3_02b0a : Inport
  State_psi_fd_SG_D_3_c9fb1 : Inport  Port=2
  State_psi_1d_SG_D_3_61581 : Inport  Port=3
  State_psi_fd_SG_D_3_fd18f : Inport  Port=4
  State_psi_1d_SG_D_3_9f27e : Inport  Port=5
  State_psi_d_SG_D_3_67b18 : Inport  Port=6
  State_psi_fd_SG_D_3_ae38b : Inport  Port=7
  State_psi_1d_SG_D_3_5274a : Inport  Port=8
  State_psi_d_SG_D_3_9355f : Inport  Port=9
  State_psi_fd_SG_D_3_ccc41 : Inport  Port=10
  Add_63540 : Sum
  Add_f1766 : Sum
  Constant_-1_bc95b : Constant  Value=-1
  Constant_-1_d3525 : Constant  Value=-1
  Constant_-1_e98ef : Constant  Value=-1
  Constant_2.0_96c98 : Constant  Value=2.0
  Constant_T_dd_696bf : Constant  Value=T_dd
  Constant_x_d_440de : Constant  Value=x_d
  Constant_x_dd_{16353,27806,28355,97144} (4 alike) : Constant  Value=x_dd
  Constant_x_dd_5c0c3 : Constant  Value=x_dd
  Constant_x_dd_b0573 : Constant  Value=x_dd
  Constant_x_dd_c5ef7 : Constant  Value=x_dd
  Constant_x_dd_debcd : Constant  Value=x_dd
  Constant_x_dd_e6d8e : Constant  Value=x_dd
  Constant_x_dd_e7920 : Constant  Value=x_dd
  Constant_x_ddd_1e697 : Constant  Value=x_ddd
  Constant_x_ddd_31e13 : Constant  Value=x_ddd
  Constant_x_ddd_7ca8a : Constant  Value=x_ddd
  Constant_x_ddd_86910 : Constant  Value=x_ddd
  Constant_x_ddd_b3c09 : Constant  Value=x_ddd
  Constant_x_ddd_c369d : Constant  Value=x_ddd
  Constant_x_ddd_f05af : Constant  Value=x_ddd
  Constant_x_l_21609 : Constant  Value=x_l
  Constant_x_l_3277b : Constant  Value=x_l
  Constant_x_l_35aa5 : Constant  Value=x_l
  Constant_x_l_35e21 : Constant  Value=x_l
  Constant_x_l_386d8 : Constant  Value=x_l
  Constant_x_l_c5f84 : Constant  Value=x_l
  Constant_x_l_f0bae : Constant  Value=x_l
  Constant_x_l_fdb3d : Constant  Value=x_l
  Divide_0fc4c : Product  Inputs=*/
  Divide_257ad : Product  Inputs=*/
  Divide_5e0ed : Product  Inputs=*/
  Divide_80eb6 : Product  Inputs=*/
  Divide_99f3b : Product  Inputs=*/
  Divide_9fde7 : Product  Inputs=*/
  Divide_b6c58 : Product  Inputs=*/
  Divide_c6b36 : Product  Inputs=*/
  Power_39c2e : Math  Operator=pow
  Product_203bf : Product
  Product_23e5b : Product
  Product_42d10 : Product
  Product_59bc2 : Product
  Product_995fd : Product
  Product_acfc8 : Product
  Product_ca87d : Product
  Product_cbee5 : Product
  Product_ed973 : Product
  Product_fcc33 : Product
  Subtract_13979 : Sum  Inputs=+-
  Subtract_31e0e : Sum  Inputs=+-
  Subtract_4345e : Sum  Inputs=+-
  Subtract_4d90e : Sum  Inputs=+-
  Subtract_5226c : Sum  Inputs=+-
  Subtract_57332 : Sum  Inputs=+-
  Subtract_57357 : Sum  Inputs=+-
  Subtract_5a44d : Sum  Inputs=+-
  Subtract_66c53 : Sum  Inputs=+-
  Subtract_6e8cf : Sum  Inputs=+-
  Subtract_7b78f : Sum  Inputs=+-
  Subtract_933f1 : Sum  Inputs=+-
  Subtract_9e7c5 : Sum  Inputs=+-
  Subtract_a0d03 : Sum  Inputs=+-
  Subtract_d342b : Sum  Inputs=+-
  Subtract_d3679 : Sum  Inputs=+-
  Subtract_d7c42 : Sum  Inputs=+-
  Subtract_e35ce : Sum  Inputs=+-
  Subtract_f26c6 : Sum  Inputs=+-
  Blockout_d_psi_fd_SG_D_3_01811 : Outport
  wires:
  Product_ca87d/1 -> Divide_80eb6/1
  Constant_-1_bc95b/1 -> Product_acfc8/1
  Subtract_57332/1 -> Product_ed973/2
  State_psi_1d_SG_D_3_9f27e/1 -> Product_acfc8/2
  Constant_x_l_3277b/1 -> Subtract_d342b/2
  Constant_x_dd_5c0c3/1 -> Subtract_57332/1
  Constant_x_ddd_c369d/1 -> Subtract_57332/2
  Product_acfc8/1 -> Product_ed973/1
  Constant_x_dd_28355/1 -> Subtract_4345e/1
  Constant_x_l_35e21/1 -> Subtract_4345e/2
  Constant_x_ddd_86910/1 -> Subtract_66c53/2
  Constant_x_ddd_f05af/1 -> Subtract_a0d03/1
  Constant_x_l_21609/1 -> Subtract_a0d03/2
  Product_42d10/1 -> Product_59bc2/1
  Product_ed973/1 -> Divide_c6b36/1
  Subtract_4345e/1 -> Divide_c6b36/2
  State_psi_fd_SG_D_3_ae38b/1 -> Product_fcc33/1
  Constant_x_ddd_1e697/1 -> Subtract_d342b/1
  Subtract_a0d03/1 -> Product_fcc33/2
  Constant_x_dd_e7920/1 -> Subtract_e35ce/1
  Constant_-1_d3525/1 -> Product_42d10/1
  Constant_x_l_fdb3d/1 -> Subtract_e35ce/2
  Product_59bc2/1 -> Divide_99f3b/1
  Divide_c6b36/1 -> Add_f1766/1
  Product_995fd/1 -> Divide_b6c58/1
  State_psi_d_SG_D_3_67b18/1 -> Add_f1766/2
  State_psi_fd_SG_D_3_ccc41/1 -> Product_995fd/1
  Product_fcc33/1 -> Divide_9fde7/1
  Constant_x_dd_97144/1 -> Subtract_f26c6/1
  Subtract_e35ce/1 -> Divide_9fde7/2
  Constant_x_l_35aa5/1 -> Subtract_6e8cf/2
  Constant_x_dd_27806/1 -> Subtract_5226c/1
  Subtract_9e7c5/1 -> Product_23e5b/2
  Constant_x_l_386d8/1 -> Subtract_5226c/2
  Divide_99f3b/1 -> Add_63540/1
  Constant_x_ddd_b3c09/1 -> Divide_80eb6/2
  Add_f1766/1 -> Subtract_57357/1
  Divide_9fde7/1 -> Subtract_57357/2
  State_psi_1d_SG_D_3_5274a/1 -> Product_42d10/2
  Constant_x_l_f0bae/1 -> Subtract_f26c6/2
  Constant_x_dd_e6d8e/1 -> Subtract_66c53/1
  Subtract_5226c/1 -> Product_ca87d/1
  Add_63540/1 -> Subtract_933f1/1
  Subtract_57357/1 -> Product_ca87d/2
  Subtract_66c53/1 -> Product_59bc2/2
  Constant_x_dd_16353/1 -> Subtract_13979/1
  Constant_x_l_c5f84/1 -> Subtract_13979/2
  Subtract_d342b/1 -> Product_995fd/2
  Constant_x_dd_debcd/1 -> Subtract_9e7c5/1
  Constant_x_ddd_7ca8a/1 -> Subtract_9e7c5/2
  Product_23e5b/1 -> Product_203bf/1
  State_psi_1d_SG_D_3_61581/1 -> Subtract_d3679/1
  Subtract_13979/1 -> Divide_99f3b/2
  State_psi_fd_SG_D_3_fd18f/1 -> Subtract_d3679/2
  Constant_-1_e98ef/1 -> Product_23e5b/1
  Subtract_d3679/1 -> Subtract_5a44d/1
  Divide_80eb6/1 -> Subtract_5a44d/2
  Constant_x_dd_c5ef7/1 -> Subtract_6e8cf/1
  Divide_b6c58/1 -> Subtract_933f1/2
  State_psi_d_SG_D_3_9355f/1 -> Add_63540/2
  Subtract_f26c6/1 -> Divide_b6c58/2
  Subtract_5a44d/1 -> Product_203bf/2
  Subtract_6e8cf/1 -> Power_39c2e/1
  Constant_2.0_96c98/1 -> Power_39c2e/2
  Product_203bf/1 -> Divide_0fc4c/1
  Subtract_d7c42/1 -> Product_cbee5/2
  Power_39c2e/1 -> Divide_0fc4c/2
  Subtract_933f1/1 -> Divide_5e0ed/1
  Constant_x_ddd_31e13/1 -> Divide_5e0ed/2
  Constant_x_d_440de/1 -> Subtract_31e0e/1
  Constant_x_dd_b0573/1 -> Subtract_31e0e/2
  Divide_0fc4c/1 -> Subtract_d7c42/1
  Divide_5e0ed/1 -> Subtract_d7c42/2
  State_E_fd_SG_D_3_02b0a/1 -> Subtract_7b78f/1
  State_psi_fd_SG_D_3_c9fb1/1 -> Subtract_7b78f/2
  Subtract_31e0e/1 -> Product_cbee5/1
  Subtract_7b78f/1 -> Subtract_4d90e/1
  Product_cbee5/1 -> Subtract_4d90e/2
  Subtract_4d90e/1 -> Divide_257ad/1
  Constant_T_dd_696bf/1 -> Divide_257ad/2
  Divide_257ad/1 -> Blockout_d_psi_fd_SG_D_3_01811/1
